simulink model "aero421_finalProjectSim0x2810x29"  (R2023b)
settings: Solver=FixedStepAuto  StartTime=0.0  StopTime=5*Period  FixedStep=10  RelTol=1e-3
values from neighbouring files (symbols this model uses):
  E0 = [phi0;theta0;psi0]    [aero421_finalProject.m]    (also in aero421_finalProject_D.m)
  q0 = [n0;e0]    [aero421_finalProject.m]    (also in aero421_finalProject_D.m)
undefined symbols (not defined in the file or in its folder): mehielSat, r_ECI_0, v_ECI_0
settings Model: Creator=emehiel  LastModifiedBy=davey
settings SolverCC: AlgebraicLoopSolver=TrustRegion
settings DebuggingCC: UnconnectedInputMsg=warning  UnconnectedOutputMsg=warning  UnconnectedLineMsg=warning
settings ModelReferenceCC: EnableRefExpFcnMdlSchedulingChecks=on

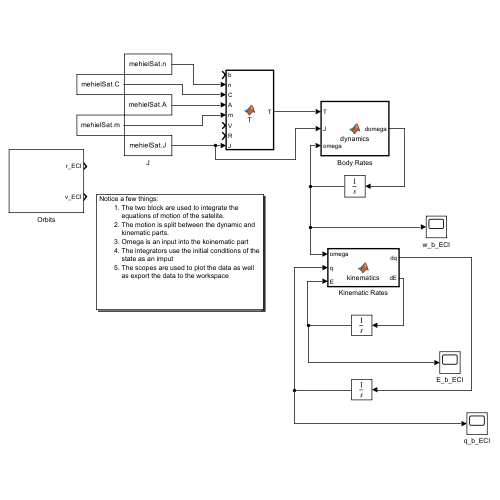
[thumbnail: Simulink's stored preview of the top-level diagram]
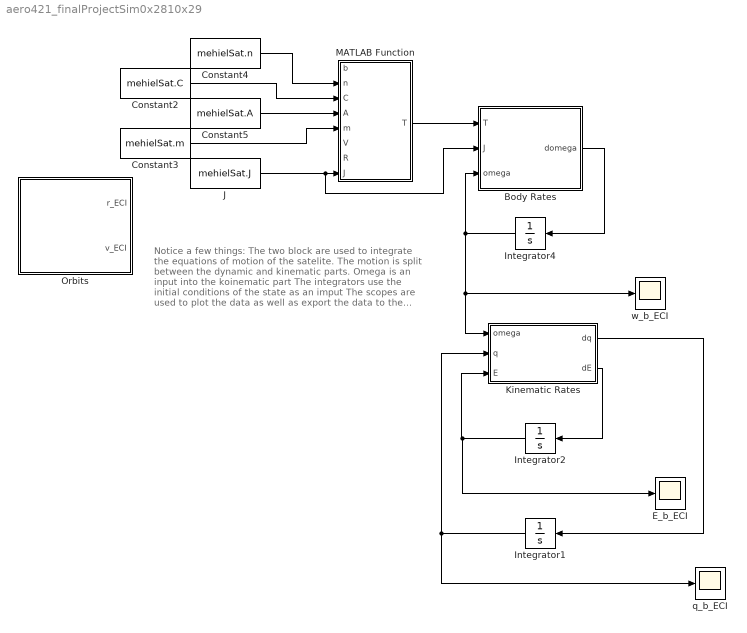
== system aero421_finalProjectSim0x2810x29 ==
  note: Notice a few things:
      | The two block are used to integrate the equations of motion of the satelite.
      | The motion is split between the dynamic and kinematic parts.
      | Omega is an input into the koinematic part
      | The integrators use the initial conditions of the state as an imput
      | The scopes are used to plot the data as well as export the data to the workspace
  Body Rates : MATLAB Function  TreatAsAtomicUnit=on
  Constant2 : Constant  Value=mehielSat.C
  Constant3 : Constant  Value=mehielSat.m
  Constant4 : Constant  Value=mehielSat.n
  Constant5 : Constant  Value=mehielSat.A
  E_b_ECI : Scope
  Integrator1 : Integrator  InitialCondition=q0
  Integrator2 : Integrator  InitialCondition=E0
  Integrator4 : Integrator  InitialCondition=mehielSat.w0
  J : Constant  Value=mehielSat.J
  Kinematic Rates : MATLAB Function  TreatAsAtomicUnit=on
  MATLAB Function : MATLAB Function  TreatAsAtomicUnit=on
  Orbits : Subsystem
  q_b_ECI : Scope
  w_b_ECI : Scope
  wires:
  MATLAB Function/1(T) -> Body Rates/1(T)
  J/1 -> Body Rates/2(J), MATLAB Function/8(J)
  Body Rates/1(domega) -> Integrator4/1
  Integrator4/1 -> Body Rates/3(omega), w_b_ECI/1, Kinematic Rates/1(omega)
  Integrator2/1 -> E_b_ECI/1, Kinematic Rates/3(E)
  Integrator1/1 -> q_b_ECI/1, Kinematic Rates/2(q)
  Kinematic Rates/2(dE) -> Integrator2/1
  Kinematic Rates/1(dq) -> Integrator1/1
  Constant4/1 -> MATLAB Function/2(n)
  Constant5/1 -> MATLAB Function/4(A)
  Constant3/1 -> MATLAB Function/5(m)
  Constant2/1 -> MATLAB Function/3(C)

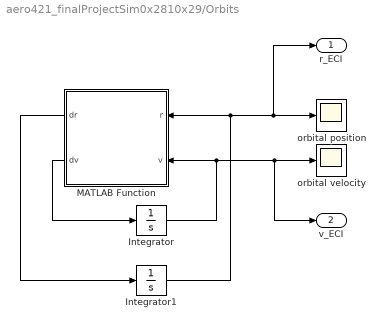
== system aero421_finalProjectSim0x2810x29/Orbits ==
  Integrator : Integrator  InitialCondition=v_ECI_0
  Integrator1 : Integrator  InitialCondition=r_ECI_0
  MATLAB Function : MATLAB Function  TreatAsAtomicUnit=on
  orbital position : Scope
  orbital velocity : Scope
  r_ECI : Outport  VectorParamsAs1DForOutWhenUnconnected=off
  v_ECI : Outport  Port=2  VectorParamsAs1DForOutWhenUnconnected=off
  wires:
  Integrator/1 -> v_ECI/1, orbital velocity/1, MATLAB Function/2(v)
  Integrator1/1 -> r_ECI/1, orbital position/1, MATLAB Function/1(r)
  MATLAB Function/1(dr) -> Integrator1/1
  MATLAB Function/2(dv) -> Integrator/1

== matlab function aero421_finalProjectSim0x2810x29/Orbits/MATLAB Function ==
  data: r input; dr output; v input; dv output
function [dr,dv] = orbitalDynamics(r, v)
%#codegen

== matlab function aero421_finalProjectSim0x2810x29/MATLAB Function ==
  data: b input; n input; C input; A input; m input; V input; R input; J input; T output
function T = T(b,n,C,A,m,V,R,J)

T = 0;
return

% Atmospherice Drag Torgue
Ta = 0;

v = norm(V);

vhat = V./v;

D = 0; % ???????

for i = 1:16
    if dot(sat.n(i,:),vhat) < 0
        continue
    end

    Cp = sat.c(i,:);
    Fa = 1/2 * D * v^2 * 2.5 * sat.A(i,:) * vhat;
    Ta = Ta + cross(Cp,Fa);
end

% Magnetic Field Torque
Tb = cross(m,b);

% Solar Pressure Torque
p = 4.5e-6;

for i = 1:16
    if dot(sat.n(i,:),s) < 0
        continue
    end

    Cp = sat.C(i,:);
    Fa = -p * s * sat.A(i,:);
    Ts = Ts + cross(Cp,Fa);
end

% Gravity Gradient Torque
rb = R; % :(

rx = vect2cross(rb);
Tg = ((3 * mu) / norm(rb)^5) * rx * J * rb;

% Total Torque
T = Ta + Tb + Ts + Tg;

T = 0;

function ax = vect2cross(a)

ax = [0 -a(3) a(2); a(3) 0 -a(1); -a(2) a(1) 0];

end

end

== matlab function aero421_finalProjectSim0x2810x29/Kinematic Rates ==
  data: omega input; q input; dq output; E input; dE output
function [dq,dE] = kinematics(omega, q, E)
%#codegen

% unpack quaternion

% compute the derivative of the quaternion components here

% compute the derivative of the Euler Angle components here


% The spacecraft initial attitude is such that it is aligned with F_LVLH
% Compute initial quaternion and EULER angles relating Fb and Feci

n = q(1)
e = q(2:4)

dn =-1/2 * e' * omega
de = 1/2 * (n * eye(3) + vect2cross(e)) * omega

dq = [dn; de];

phi   = E(1);
theta = E(2);

dE = [1, sin(phi)*tan(theta), cos(phi)*tan(theta); ...
     0, cos(phi)           ,-sin(phi);            ...
     0, sin(phi)*sec(theta), cos(phi)*sec(theta)] * omega;

end

== matlab function aero421_finalProjectSim0x2810x29/Body Rates ==
  data: T input; J input; omega input; domega output
function domega = dynamics(T, J, omega)
%#codegen

% Compute the derivative of the angular velocity $\omega$ here

% Using the Euler Equations

J = sat.J;

wXdot = (-(J(3,3)-J(2,2))*omega(2)*omega(3))/J(1,1) + T;
wYdot = (-(J(1,1)-J(3,3))*omega(1)*omega(3))/J(2,2) + T;
wZdot = (-(J(2,2)-J(1,1))*omega(1)*omega(2))/J(3,3) + T;
domega = [wXdot; wYdot; wZdot];
